simulink model "Sat02"  (Simulink 7.7)
settings: Solver=ode3  StartTime=0.0  StopTime=20  FixedStep=1/100  RelTol=1e-3
values from neighbouring files (symbols this model uses):
  A = [0 1 0 0;3*omega^2 0 0 2*d*omega ... (first row only)    [insat02.m]
  B = [0 0;1 0;0 0;0 1/d^2]    [insat02.m]
  C = eye(4,4)    [insat02.m]
  cin = [.8 0 0 1]    [insat02.m]
  d = 1    [insat02.m]
  D = zeros(4,2)    [insat02.m]
  H = [1 0 0 0;0 0 1 0]    [insat02.m]
  omega = 1    [insat02.m]
undefined symbols (not defined in the file or in its folder): K
libraries: simulink x3
settings Model: Creator=user  LastModifiedBy=Vargas
settings DataIOCC: SignalLoggingName=sigsOut
settings OptimizationCC: InitFltsAndDblsToZero=on
settings DebuggingCC: SaveWithParameterizedLinksMsg=none  SignalResolutionControl=TryResolveAllWithWarning  SolverPrmCheckMsg=none  MultiTaskDSMMsg=warning  MultiTaskCondExecSysMsg=none  StrictBusMsg=None
settings HardwareCC: TargetUnknown=on
settings RTWCC: IncludeERTFirstTime=on
settings GRTTargetCC: ModelReferenceCompliant=off  CompOptLevelCompliant=off  MatFileLogging=off

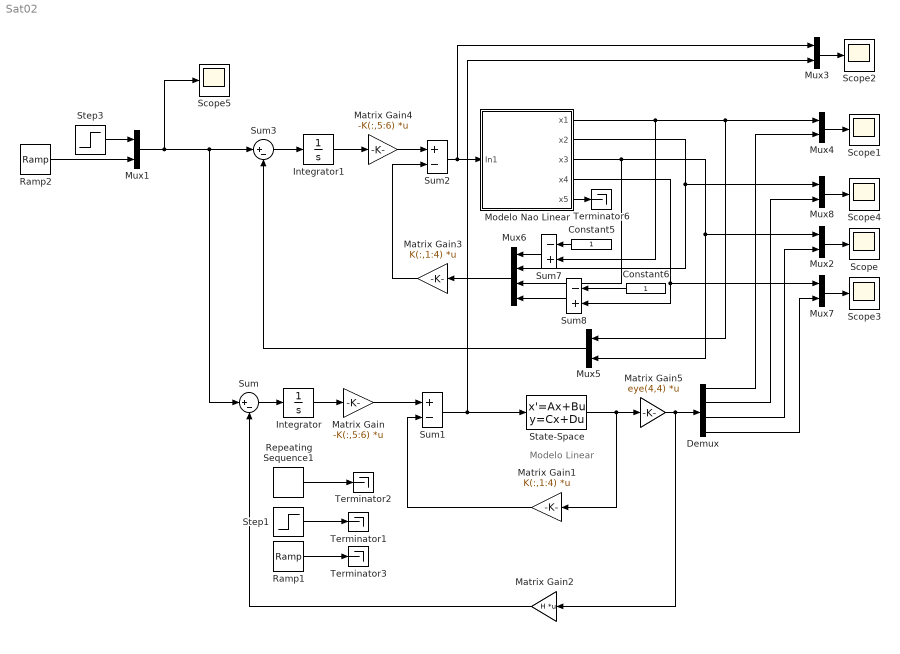
== system Sat02 ==
  note: Modelo Linear
  Constant5 : Constant
  Constant6 : Constant
  Demux : Demux
  Integrator : Integrator
  Integrator1 : Integrator
  Matrix Gain : Gain  Gain=-K(:,5:6)  Multiplication=Matrix(K*u)  SaturateOnIntegerOverflow=on  OutDataTypeStr=Inherit: Same as input  ParamDataTypeStr=Inherit: Same as input
  Matrix Gain1 : Gain  Gain=K(:,1:4)  Multiplication=Matrix(K*u)  SaturateOnIntegerOverflow=on  OutDataTypeStr=Inherit: Same as input  ParamDataTypeStr=Inherit: Same as input
  Matrix Gain2 : Gain  Gain=H  Multiplication=Matrix(K*u)  SaturateOnIntegerOverflow=on  OutDataTypeStr=Inherit: Same as input  ParamDataTypeStr=Inherit: Same as input
  Matrix Gain3 : Gain  Gain=K(:,1:4)  Multiplication=Matrix(K*u)  SaturateOnIntegerOverflow=on  OutDataTypeStr=Inherit: Same as input  ParamDataTypeStr=Inherit: Same as input
  Matrix Gain4 : Gain  Gain=-K(:,5:6)  Multiplication=Matrix(K*u)  SaturateOnIntegerOverflow=on  OutDataTypeStr=Inherit: Same as input  ParamDataTypeStr=Inherit: Same as input
  Matrix Gain5 : Gain  Gain=eye(4,4)  Multiplication=Matrix(K*u)  SaturateOnIntegerOverflow=on  OutDataTypeStr=Inherit: Same as input  ParamDataTypeStr=Inherit: Same as input
  Modelo Nao Linear : Subsystem
      mask Display: image(imread('earth-with-satellite.png'))
  Mux{1..5,7..8} (7 alike) : Mux  Inputs=2
  Mux6 : Mux
  Ramp1 : simulink/Sources/Ramp  SystemSampleTime=-1  slope=0.5  start=0  X0=0
  Ramp2 : simulink/Sources/Ramp  SystemSampleTime=-1  slope=0.5  start=0  X0=0
  Repeating Sequence1 : simulink/Sources/Repeating Sequence  SystemSampleTime=-1  rep_seq_t=[0 5 15 30 40 60]  rep_seq_y=[0 0 1 1 0 0]
  Scope{,1..5} (6 alike) : Scope
      Scope settings: TimeRange=20  YMin=0  YMax=10  SaveName=ScopeData3  DataFormat=Array
      Scope1 settings: TimeRange=20  YMin=-0.0125  YMax=0.03  DataFormat=Array
      Scope2 settings: YMin=-0.1  YMax=0.1  SaveName=ScopeData5  DataFormat=Array
      Scope3 settings: YMin=-0.1  YMax=0.1  SaveName=ScopeData4  DataFormat=Array
      Scope4 settings: YMin=-0.1  YMax=0.1  SaveName=ScopeData2  DataFormat=Array
      Scope5 settings: YMin=-0.1  YMax=0.1  SaveName=ScopeData6  DataFormat=Array
  State-Space : StateSpace  A=A  B=B  C=C  D=D  X0=cin
  Step1 : Step  Time=0  After=pi/4  SampleTime=0
  Step3 : Step  Time=0  SampleTime=0
  Sum : Sum  Inputs=|+-  SaturateOnIntegerOverflow=on
  Sum1 : Sum  Inputs=+-  SaturateOnIntegerOverflow=on
  Sum2 : Sum  Inputs=+-  SaturateOnIntegerOverflow=on
  Sum3 : Sum  Inputs=|+-  SaturateOnIntegerOverflow=on
  Sum7 : Sum  Inputs=-+  SaturateOnIntegerOverflow=on
  Sum8 : Sum  Inputs=-+  SaturateOnIntegerOverflow=on
  Terminator{1..3,6} (4 alike) : Terminator
  wires:
  Sum2/1 -> Modelo Nao Linear/1(In1), Mux3/1
  Integrator1/1 -> Matrix Gain4/1
  Mux1/1 -> Sum/1, Sum3/1, Scope5/1
  Sum3/1 -> Integrator1/1
  Modelo Nao Linear/4(x4) -> Sum8/2, Mux7/1
  Modelo Nao Linear/2(x2) -> Mux6/2, Mux8/1
  State-Space/1 -> Matrix Gain1/1, Matrix Gain5/1
  Sum1/1 -> State-Space/1, Mux3/2
  Integrator/1 -> Matrix Gain/1
  Sum/1 -> Integrator/1
  Matrix Gain1/1 -> Sum1/2
  Step1/1 -> Terminator1/1
  Repeating Sequence1/1 -> Terminator2/1
  Matrix Gain5/1 -> Demux/1, Matrix Gain2/1
  Ramp1/1 -> Terminator3/1
  Mux3/1 -> Scope2/1
  Mux4/1 -> Scope1/1
  Modelo Nao Linear/1(x1) -> Mux4/1, Mux5/1, Sum7/2
  Matrix Gain/1 -> Sum1/1
  Matrix Gain3/1 -> Sum2/2
  Matrix Gain4/1 -> Sum2/1
  Ramp2/1 -> Mux1/2
  Step3/1 -> Mux1/1
  Mux5/1 -> Sum3/2
  Modelo Nao Linear/3(x3) -> Mux6/3, Mux5/2, Mux2/1
  Constant5/1 -> Sum7/1
  Constant6/1 -> Sum8/1
  Sum7/1 -> Mux6/1
  Sum8/1 -> Mux6/4
  Mux6/1 -> Matrix Gain3/1
  Modelo Nao Linear/5(x5) -> Terminator6/1
  Mux2/1 -> Scope/1
  Mux7/1 -> Scope3/1
  Matrix Gain2/1 -> Sum/2
  Demux/1 -> Mux4/2
  Demux/2 -> Mux8/2
  Demux/3 -> Mux2/2
  Demux/4 -> Mux7/2
  Mux8/1 -> Scope4/1

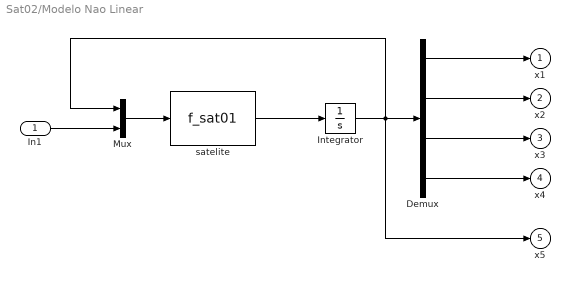
== system Sat02/Modelo Nao Linear ==
  In1 : Inport
  Demux : Demux
  Integrator : Integrator  InitialCondition=cin
  Mux : Mux  Inputs=2
  satelite : S-Function  FunctionName=f_sat01  Parameters=omega,d  EnableBusSupport=off
  x1 : Outport
  x2 : Outport  Port=2
  x3 : Outport  Port=3
  x4 : Outport  Port=4
  x5 : Outport  Port=5
  wires:
  Demux/1 -> x1/1
  Demux/2 -> x2/1
  satelite/1 -> Integrator/1
  Integrator/1 -> Demux/1, x5/1, Mux/1
  Mux/1 -> satelite/1
  Demux/3 -> x3/1
  Demux/4 -> x4/1
  In1/1 -> Mux/2
